simulink model "maglevAGH_Luenberger"  (R2020a)
settings: Solver=ode45  StartTime=0.0  StopTime=5  MaxStep=0.001  RelTol=1e-3  EnableMultiTasking=on
values from neighbouring files (symbols this model uses):
  A = [0, 1, 0 ... (first row only)    [identification_data.m]
  B = [0; 0; 1/L_ep]    [identification_data.m]
  C = [1 0 0; 0 0 1]    [identification_data.m]
  g_E = 9.81    [identification_data.m]
  i_ep = sqrt(-2*m_b*g_E/L_d_ep)    [identification_data.m]
  K_lq = lqr(A,B,Q,R)    [identification_data.m]
  L = place(A',C',pp)'    [identification_data.m]
  m_b = 58e-3    (= 0.058)    [identification_data.m]
  R_n = mean(R(1:end-1))    [identification_data.m]
  u_ep = R_n * i_ep    [identification_data.m]
  z_ep = 0.010    (= 0.01)    [identification_data.m]
undefined symbols (not defined in the file or in its folder): ind
settings Model: Creator=tutaj  LastModifiedBy=wkula
settings DataIOCC: LimitDataPoints=on  SaveFormat=Array  ReturnWorkspaceOutputs=off
settings OptimizationCC: LifeSpan=inf
settings DebuggingCC: UnderspecifiedInitializationDetection=Classic  MergeDetectMultiDrivingBlocksExec=none  SolverPrmCheckMsg=warning  StateNameClashWarn=warning  SFUnexpectedBacktrackingDiag=warning  SFNoUnconditionalDefaultTransitionDiag=warning  SFExecutionAtInitializationDiag=none  ArithmeticOperatorsInVariantConditions=warning
settings HardwareCC: ProdBitPerPointer=32  ProdBitPerSizeT=32  ProdBitPerPtrDiffT=32  ProdLargestAtomicFloat=None  ProdIntDivRoundTo=Undefined  ProdEndianess=Unspecified  ProdWordSize=32  ProdHWDeviceType=32-bit Generic
settings ModelReferenceCC: PropagateSignalLabelsOutOfModel=off
settings SFSimCC: SimUseLocalCustomCode=off  CustomCodeUndefinedFunction=UseInterfaceOnly
settings RTWCC: RTWUseLocalCustomCode=off
settings CodeAppCC: StateflowObjectComments=on
settings GRTTargetCC: TargetLangStandard=C89/C90 (ANSI)
settings ConfigComp: CovMetricSettings=dw  CovHtmlReporting=on  CovSaveCumulativeToWorkspaceVar=on  CovSaveSingleToWorkspaceVar=on  CovExternalEMLEnable=off

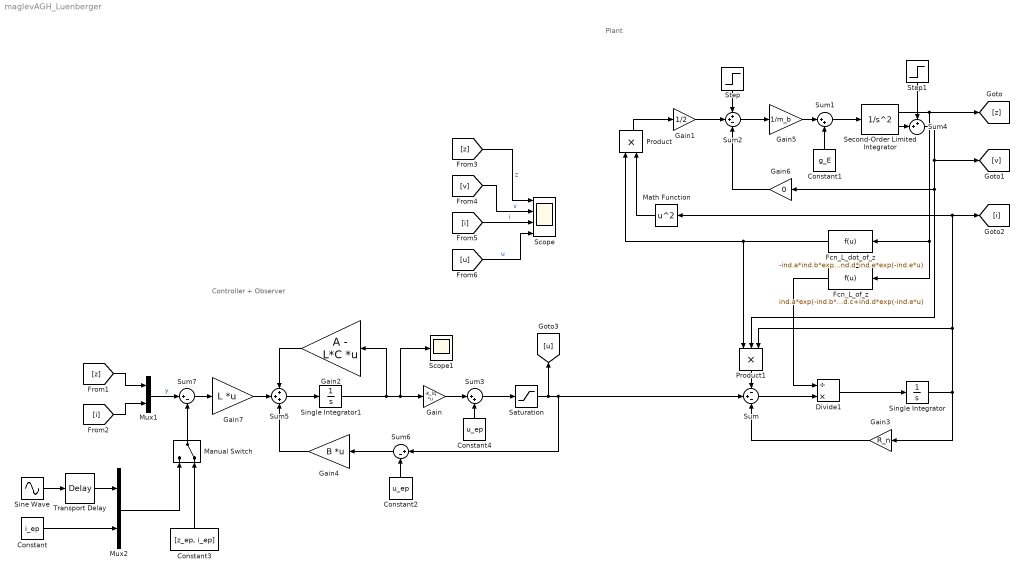
== system maglevAGH_Luenberger ==
  note: Controller + Observer
  note: Plant
  Constant : Constant  Value=i_ep
  Constant1 : Constant  Value=g_E
  Constant2 : Constant  Value=u_ep
  Constant3 : Constant  Value=[z_ep, i_ep]
  Constant4 : Constant  Value=u_ep
  Divide1 : Product  Inputs=/*
  Fcn_L_dot_of_z : Fcn  Expr=-ind.a*ind.b*exp(-ind.b*u)-ind.d*ind.e*exp(-ind.e*u)
  Fcn_L_of_z : Fcn  Expr=ind.a*exp(-ind.b*u)+ind.c+ind.d*exp(-ind.e*u)
  Gain : Gain  Gain=-K_lq  Multiplication=Matrix(K*u) (u vector)
  Gain1 : Gain  Gain=1/2
  Gain2 : Gain  Gain=A - L*C  Multiplication=Matrix(K*u) (u vector)
  Gain3 : Gain  Gain=R_n
  Gain4 : Gain  Gain=B  Multiplication=Matrix(K*u) (u vector)
  Gain5 : Gain  Gain=1/m_b
  Gain6 : Gain  Gain=0
  Gain7 : Gain  Gain=L  Multiplication=Matrix(K*u) (u vector)
  Manual Switch : ManualSwitch  CurrentSetting=0
  Math Function : Math  Operator=square  SignedPower=on  SaturateOnIntegerOverflow=on
  Mux1 : Mux  Inputs=2
  Mux2 : Mux  Inputs=2
  Product : Product
  Product1 : Product  Inputs=3
  Saturation : Saturate  UpperLimit=12  LowerLimit=0
  Scope : Scope  NumInputPorts=4
  Scope1 : Scope
  Second-Order Limited Integrator : SecondOrderIntegrator  ICX=z_ep  LimitX=on  UpperLimitX=0.2  LowerLimitX=0  ICDXDT=v_ep
  Sine Wave : Sin  Amplitude=0.008  Bias=z_ep  SampleTime=0
  Single Integrator : Integrator  InitialCondition=i_ep
  Single Integrator1 : Integrator
  Step : Step  Time=2  After=0  SampleTime=0
  Step1 : Step  Time=2  After=0.001  SampleTime=0
  Sum : Sum  Inputs=-+-
  Sum1 : Sum  Inputs=|++
  Sum2 : Sum  Inputs=++-
  Sum3 : Sum  Inputs=|++
  Sum4 : Sum  Inputs=++|
  Sum5 : Sum  Inputs=+++
  Sum6 : Sum  Inputs=|+-
  Sum7 : Sum  Inputs=|+-
  Transport Delay : TransportDelay
  wires:
  Gain6/1 -> Sum2/3
  Gain7/1 -> Sum5/2
  [i] -> Scope/3  "i"
  Gain2/1 -> Sum5/1
  Sum7/1 -> Gain7/1
  Saturation/1 -> [u], Sum6/1, Sum/2
  Constant2/1 -> Sum6/2
  Divide1/1 -> Single Integrator/1
  Sum3/1 -> Saturation/1
  [z] -> Scope/1  "z"
  Constant4/1 -> Sum3/2
  [z] -> Mux1/1
  [u] -> Scope/4  "u"
  [v] -> Scope/2  "v"
  Mux1/1 -> Sum7/1  "y"
  Sum/1 -> Divide1/2
  Gain4/1 -> Sum5/3
  Sum5/1 -> Single Integrator1/1
  Single Integrator/1 -> Gain3/1, Math Function/1, [i], Product1/3
  Sum2/1 -> Gain5/1
  Gain5/1 -> Sum1/1
  Constant1/1 -> Sum1/2
  Product1/1 -> Sum/1
  Fcn_L_of_z/1 -> Divide1/1
  Fcn_L_dot_of_z/1 -> Product/1, Product1/1
  Single Integrator1/1 -> Gain/1, Scope1/1, Gain2/1
  Gain3/1 -> Sum/3
  Sum4/1 -> [v], Product1/2, Gain6/1
  Sum1/1 -> Second-Order Limited Integrator/1
  [i] -> Mux1/2
  Gain1/1 -> Sum2/2
  Product/1 -> Gain1/1
  Gain/1 -> Sum3/1
  Math Function/1 -> Product/2
  Sum6/1 -> Gain4/1
  Second-Order Limited Integrator/1 -> [z], Fcn_L_dot_of_z/1, Fcn_L_of_z/1
  Constant/1 -> Mux2/2
  Sine Wave/1 -> Transport Delay/1
  Transport Delay/1 -> Mux2/1
  Manual Switch/1 -> Sum7/2
  Mux2/1 -> Manual Switch/1
  Constant3/1 -> Manual Switch/2
  Step/1 -> Sum2/1
  Step1/1 -> Sum4/1
  Second-Order Limited Integrator/2 -> Sum4/2
